simulink library "r2daq_blocks"  (R2012b)
settings: Solver=ode45  StartTime=0.0  StopTime=10.0  RelTol=1e-3
undefined symbols (not defined in the file or in its folder): biquad_iir, feedback_iir, filters, libddc, sfp, synth, xlfir_8x16
libraries: xbsIndex_r4 x4088, casper_library_misc x21, dspsigops x16, casper_library_delays x10, xps_library x1
(part 5 of 23)

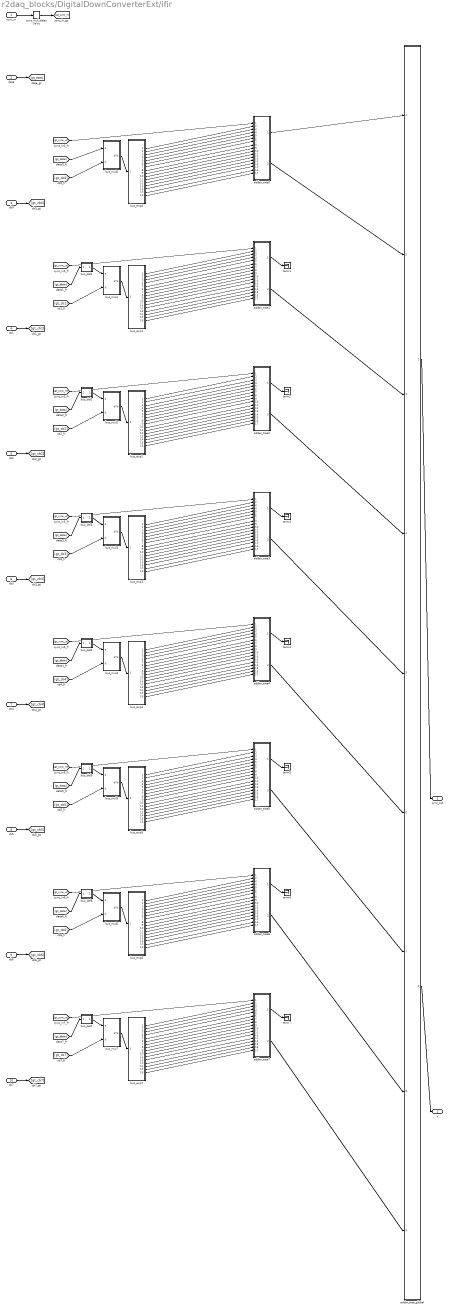
== system r2daq_blocks/DigitalDownConverterExt/ifir ==
  sync_in : Inport
  data : Inport  Port=2
  cb0 : Inport  Port=3
  cb1 : Inport  Port=4
  cb2 : Inport  Port=5
  cb3 : Inport  Port=6
  cb4 : Inport  Port=7
  cb5 : Inport  Port=8
  cb6 : Inport  Port=9
  cb7 : Inport  Port=10
  adder_tree0 : Subsystem  AncestorBlock=casper_library_misc/adder_tree  mask(adder_tree){n_inputs=16, latency=1, adder_imp=Fabric, first_stage_hdl=on}
      mask prompts: n_inputs "Number of Inputs"; latency "Add Latency"; adder_imp "Adder implementation"; first_stage_hdl "Use behavioural HDL for first stage of adders"
      mask help:
      | Sums all inputs using a tree of adds and delays.
      |
      | Number of inputs: The number of inputs to the block to be summed
      | Add latency: The number of clock cycles to perform one addition (affects timing)..
      | Adder implementation: choice of fabric or DSP48E core, or behavioral HDL
      | Use behavioural HDL for first stage of adders: Causes the first stage of adders to be absorbed into DSP blocks if multipliers precede them (Virtex 5). Overrides Adder implementation
      mask init:
      | adder_tree_init(gcb, ...
      |     'n_inputs', n_inputs, ...
      |     'latency', latency, ...
      |     'adder_imp', adder_imp, ...
      |     'first_stage_hdl', first_stage_hdl);
      settings: AttributesFormatString=latency 4
      mask Help: eval('xlWeb(''http://casper.berkeley.edu/wiki/Adder_tree'')')
      mask TypeOptions adder_imp: Behavioral | Fabric | DSP48
  adder_tree1 : Subsystem  AncestorBlock=casper_library_misc/adder_tree  mask(adder_tree){n_inputs=16, latency=1, adder_imp=Fabric, first_stage_hdl=on}
      mask prompts: n_inputs "Number of Inputs"; latency "Add Latency"; adder_imp "Adder implementation"; first_stage_hdl "Use behavioural HDL for first stage of adders"
      mask help:
      | Sums all inputs using a tree of adds and delays.
      |
      | Number of inputs: The number of inputs to the block to be summed
      | Add latency: The number of clock cycles to perform one addition (affects timing)..
      | Adder implementation: choice of fabric or DSP48E core, or behavioral HDL
      | Use behavioural HDL for first stage of adders: Causes the first stage of adders to be absorbed into DSP blocks if multipliers precede them (Virtex 5). Overrides Adder implementation
      mask init:
      | adder_tree_init(gcb, ...
      |     'n_inputs', n_inputs, ...
      |     'latency', latency, ...
      |     'adder_imp', adder_imp, ...
      |     'first_stage_hdl', first_stage_hdl);
      settings: AttributesFormatString=latency 4
      mask Help: eval('xlWeb(''http://casper.berkeley.edu/wiki/Adder_tree'')')
      mask TypeOptions adder_imp: Behavioral | Fabric | DSP48
  adder_tree2 : Subsystem  AncestorBlock=casper_library_misc/adder_tree  mask(adder_tree){n_inputs=16, latency=1, adder_imp=Fabric, first_stage_hdl=on}
      mask prompts: n_inputs "Number of Inputs"; latency "Add Latency"; adder_imp "Adder implementation"; first_stage_hdl "Use behavioural HDL for first stage of adders"
      mask help:
      | Sums all inputs using a tree of adds and delays.
      |
      | Number of inputs: The number of inputs to the block to be summed
      | Add latency: The number of clock cycles to perform one addition (affects timing)..
      | Adder implementation: choice of fabric or DSP48E core, or behavioral HDL
      | Use behavioural HDL for first stage of adders: Causes the first stage of adders to be absorbed into DSP blocks if multipliers precede them (Virtex 5). Overrides Adder implementation
      mask init:
      | adder_tree_init(gcb, ...
      |     'n_inputs', n_inputs, ...
      |     'latency', latency, ...
      |     'adder_imp', adder_imp, ...
      |     'first_stage_hdl', first_stage_hdl);
      settings: AttributesFormatString=latency 4
      mask Help: eval('xlWeb(''http://casper.berkeley.edu/wiki/Adder_tree'')')
      mask TypeOptions adder_imp: Behavioral | Fabric | DSP48
  adder_tree3 : Subsystem  AncestorBlock=casper_library_misc/adder_tree  mask(adder_tree){n_inputs=16, latency=1, adder_imp=Fabric, first_stage_hdl=on}
      mask prompts: n_inputs "Number of Inputs"; latency "Add Latency"; adder_imp "Adder implementation"; first_stage_hdl "Use behavioural HDL for first stage of adders"
      mask help:
      | Sums all inputs using a tree of adds and delays.
      |
      | Number of inputs: The number of inputs to the block to be summed
      | Add latency: The number of clock cycles to perform one addition (affects timing)..
      | Adder implementation: choice of fabric or DSP48E core, or behavioral HDL
      | Use behavioural HDL for first stage of adders: Causes the first stage of adders to be absorbed into DSP blocks if multipliers precede them (Virtex 5). Overrides Adder implementation
      mask init:
      | adder_tree_init(gcb, ...
      |     'n_inputs', n_inputs, ...
      |     'latency', latency, ...
      |     'adder_imp', adder_imp, ...
      |     'first_stage_hdl', first_stage_hdl);
      settings: AttributesFormatString=latency 4
      mask Help: eval('xlWeb(''http://casper.berkeley.edu/wiki/Adder_tree'')')
      mask TypeOptions adder_imp: Behavioral | Fabric | DSP48
  adder_tree4 : Subsystem  AncestorBlock=casper_library_misc/adder_tree  mask(adder_tree){n_inputs=16, latency=1, adder_imp=Fabric, first_stage_hdl=on}
      mask prompts: n_inputs "Number of Inputs"; latency "Add Latency"; adder_imp "Adder implementation"; first_stage_hdl "Use behavioural HDL for first stage of adders"
      mask help:
      | Sums all inputs using a tree of adds and delays.
      |
      | Number of inputs: The number of inputs to the block to be summed
      | Add latency: The number of clock cycles to perform one addition (affects timing)..
      | Adder implementation: choice of fabric or DSP48E core, or behavioral HDL
      | Use behavioural HDL for first stage of adders: Causes the first stage of adders to be absorbed into DSP blocks if multipliers precede them (Virtex 5). Overrides Adder implementation
      mask init:
      | adder_tree_init(gcb, ...
      |     'n_inputs', n_inputs, ...
      |     'latency', latency, ...
      |     'adder_imp', adder_imp, ...
      |     'first_stage_hdl', first_stage_hdl);
      settings: AttributesFormatString=latency 4
      mask Help: eval('xlWeb(''http://casper.berkeley.edu/wiki/Adder_tree'')')
      mask TypeOptions adder_imp: Behavioral | Fabric | DSP48
  adder_tree5 : Subsystem  AncestorBlock=casper_library_misc/adder_tree  mask(adder_tree){n_inputs=16, latency=1, adder_imp=Fabric, first_stage_hdl=on}
      mask prompts: n_inputs "Number of Inputs"; latency "Add Latency"; adder_imp "Adder implementation"; first_stage_hdl "Use behavioural HDL for first stage of adders"
      mask help:
      | Sums all inputs using a tree of adds and delays.
      |
      | Number of inputs: The number of inputs to the block to be summed
      | Add latency: The number of clock cycles to perform one addition (affects timing)..
      | Adder implementation: choice of fabric or DSP48E core, or behavioral HDL
      | Use behavioural HDL for first stage of adders: Causes the first stage of adders to be absorbed into DSP blocks if multipliers precede them (Virtex 5). Overrides Adder implementation
      mask init:
      | adder_tree_init(gcb, ...
      |     'n_inputs', n_inputs, ...
      |     'latency', latency, ...
      |     'adder_imp', adder_imp, ...
      |     'first_stage_hdl', first_stage_hdl);
      settings: AttributesFormatString=latency 4
      mask Help: eval('xlWeb(''http://casper.berkeley.edu/wiki/Adder_tree'')')
      mask TypeOptions adder_imp: Behavioral | Fabric | DSP48
  adder_tree6 : Subsystem  AncestorBlock=casper_library_misc/adder_tree  mask(adder_tree){n_inputs=16, latency=1, adder_imp=Fabric, first_stage_hdl=on}
      mask prompts: n_inputs "Number of Inputs"; latency "Add Latency"; adder_imp "Adder implementation"; first_stage_hdl "Use behavioural HDL for first stage of adders"
      mask help:
      | Sums all inputs using a tree of adds and delays.
      |
      | Number of inputs: The number of inputs to the block to be summed
      | Add latency: The number of clock cycles to perform one addition (affects timing)..
      | Adder implementation: choice of fabric or DSP48E core, or behavioral HDL
      | Use behavioural HDL for first stage of adders: Causes the first stage of adders to be absorbed into DSP blocks if multipliers precede them (Virtex 5). Overrides Adder implementation
      mask init:
      | adder_tree_init(gcb, ...
      |     'n_inputs', n_inputs, ...
      |     'latency', latency, ...
      |     'adder_imp', adder_imp, ...
      |     'first_stage_hdl', first_stage_hdl);
      settings: AttributesFormatString=latency 4
      mask Help: eval('xlWeb(''http://casper.berkeley.edu/wiki/Adder_tree'')')
      mask TypeOptions adder_imp: Behavioral | Fabric | DSP48
  adder_tree7 : Subsystem  AncestorBlock=casper_library_misc/adder_tree  mask(adder_tree){n_inputs=16, latency=1, adder_imp=Fabric, first_stage_hdl=on}
      mask prompts: n_inputs "Number of Inputs"; latency "Add Latency"; adder_imp "Adder implementation"; first_stage_hdl "Use behavioural HDL for first stage of adders"
      mask help:
      | Sums all inputs using a tree of adds and delays.
      |
      | Number of inputs: The number of inputs to the block to be summed
      | Add latency: The number of clock cycles to perform one addition (affects timing)..
      | Adder implementation: choice of fabric or DSP48E core, or behavioral HDL
      | Use behavioural HDL for first stage of adders: Causes the first stage of adders to be absorbed into DSP blocks if multipliers precede them (Virtex 5). Overrides Adder implementation
      mask init:
      | adder_tree_init(gcb, ...
      |     'n_inputs', n_inputs, ...
      |     'latency', latency, ...
      |     'adder_imp', adder_imp, ...
      |     'first_stage_hdl', first_stage_hdl);
      settings: AttributesFormatString=latency 4
      mask Help: eval('xlWeb(''http://casper.berkeley.edu/wiki/Adder_tree'')')
      mask TypeOptions adder_imp: Behavioral | Fabric | DSP48
  adder_tree_global : Subsystem  AncestorBlock=casper_library_misc/adder_tree  mask(adder_tree){n_inputs=8, latency=1, adder_imp=Fabric, first_stage_hdl=on}
      mask prompts: n_inputs "Number of Inputs"; latency "Add Latency"; adder_imp "Adder implementation"; first_stage_hdl "Use behavioural HDL for first stage of adders"
      mask help:
      | Sums all inputs using a tree of adds and delays.
      |
      | Number of inputs: The number of inputs to the block to be summed
      | Add latency: The number of clock cycles to perform one addition (affects timing)..
      | Adder implementation: choice of fabric or DSP48E core, or behavioral HDL
      | Use behavioural HDL for first stage of adders: Causes the first stage of adders to be absorbed into DSP blocks if multipliers precede them (Virtex 5). Overrides Adder implementation
      mask init:
      | adder_tree_init(gcb, ...
      |     'n_inputs', n_inputs, ...
      |     'latency', latency, ...
      |     'adder_imp', adder_imp, ...
      |     'first_stage_hdl', first_stage_hdl);
      settings: AttributesFormatString=latency 3
      mask Help: eval('xlWeb(''http://casper.berkeley.edu/wiki/Adder_tree'')')
      mask TypeOptions adder_imp: Behavioral | Fabric | DSP48
  bus_del1 : Subsystem  AncestorBlock=casper_library_bus/bus_delay  mask(bus_delay){n_bits=[18 18 18 18 18 18 18 18 18 18 18 18 18 18 18 18], latency=1, cmplx=off, enable=off, reg_retiming=on, misc=off}
      mask prompts: n_bits "input bit widths"; cmplx "complex data"; enable "enable port"; reg_retiming "implement using behavioral HDL"; misc "misc support"
      mask help: Delay components of a bus
      mask init:
      | bus_delay_init(gcb, ...
      |     'enable', enable, ...
      |     'cmplx', cmplx, ...
      |     'n_bits', n_bits, ...
      |     'latency', latency, ...
      |     'reg_retiming', reg_retiming, ...
      |     'misc', misc);
  bus_del2 : Subsystem  AncestorBlock=casper_library_bus/bus_delay  mask(bus_delay){n_bits=[18 18 18 18 18 18 18 18 18 18 18 18 18 18 18 18], latency=2, cmplx=off, enable=off, reg_retiming=on, misc=off}
      mask prompts: n_bits "input bit widths"; cmplx "complex data"; enable "enable port"; reg_retiming "implement using behavioral HDL"; misc "misc support"
      mask help: Delay components of a bus
      mask init:
      | bus_delay_init(gcb, ...
      |     'enable', enable, ...
      |     'cmplx', cmplx, ...
      |     'n_bits', n_bits, ...
      |     'latency', latency, ...
      |     'reg_retiming', reg_retiming, ...
      |     'misc', misc);
  bus_del3 : Subsystem  AncestorBlock=casper_library_bus/bus_delay  mask(bus_delay){n_bits=[18 18 18 18 18 18 18 18 18 18 18 18 18 18 18 18], latency=3, cmplx=off, enable=off, reg_retiming=on, misc=off}
      mask prompts: n_bits "input bit widths"; cmplx "complex data"; enable "enable port"; reg_retiming "implement using behavioral HDL"; misc "misc support"
      mask help: Delay components of a bus
      mask init:
      | bus_delay_init(gcb, ...
      |     'enable', enable, ...
      |     'cmplx', cmplx, ...
      |     'n_bits', n_bits, ...
      |     'latency', latency, ...
      |     'reg_retiming', reg_retiming, ...
      |     'misc', misc);
  bus_del4 : Subsystem  AncestorBlock=casper_library_bus/bus_delay  mask(bus_delay){n_bits=[18 18 18 18 18 18 18 18 18 18 18 18 18 18 18 18], latency=4, cmplx=off, enable=off, reg_retiming=on, misc=off}
      mask prompts: n_bits "input bit widths"; cmplx "complex data"; enable "enable port"; reg_retiming "implement using behavioral HDL"; misc "misc support"
      mask help: Delay components of a bus
      mask init:
      | bus_delay_init(gcb, ...
      |     'enable', enable, ...
      |     'cmplx', cmplx, ...
      |     'n_bits', n_bits, ...
      |     'latency', latency, ...
      |     'reg_retiming', reg_retiming, ...
      |     'misc', misc);
  bus_del5 : Subsystem  AncestorBlock=casper_library_bus/bus_delay  mask(bus_delay){n_bits=[18 18 18 18 18 18 18 18 18 18 18 18 18 18 18 18], latency=5, cmplx=off, enable=off, reg_retiming=on, misc=off}
      mask prompts: n_bits "input bit widths"; cmplx "complex data"; enable "enable port"; reg_retiming "implement using behavioral HDL"; misc "misc support"
      mask help: Delay components of a bus
      mask init:
      | bus_delay_init(gcb, ...
      |     'enable', enable, ...
      |     'cmplx', cmplx, ...
      |     'n_bits', n_bits, ...
      |     'latency', latency, ...
      |     'reg_retiming', reg_retiming, ...
      |     'misc', misc);
  bus_del6 : Subsystem  AncestorBlock=casper_library_bus/bus_delay  mask(bus_delay){n_bits=[18 18 18 18 18 18 18 18 18 18 18 18 18 18 18 18], latency=6, cmplx=off, enable=off, reg_retiming=on, misc=off}
      mask prompts: n_bits "input bit widths"; cmplx "complex data"; enable "enable port"; reg_retiming "implement using behavioral HDL"; misc "misc support"
      mask help: Delay components of a bus
      mask init:
      | bus_delay_init(gcb, ...
      |     'enable', enable, ...
      |     'cmplx', cmplx, ...
      |     'n_bits', n_bits, ...
      |     'latency', latency, ...
      |     'reg_retiming', reg_retiming, ...
      |     'misc', misc);
  bus_del7 : Subsystem  AncestorBlock=casper_library_bus/bus_delay  mask(bus_delay){n_bits=[18 18 18 18 18 18 18 18 18 18 18 18 18 18 18 18], latency=7, cmplx=off, enable=off, reg_retiming=on, misc=off}
      mask prompts: n_bits "input bit widths"; cmplx "complex data"; enable "enable port"; reg_retiming "implement using behavioral HDL"; misc "misc support"
      mask help: Delay components of a bus
      mask init:
      | bus_delay_init(gcb, ...
      |     'enable', enable, ...
      |     'cmplx', cmplx, ...
      |     'n_bits', n_bits, ...
      |     'latency', latency, ...
      |     'reg_retiming', reg_retiming, ...
      |     'misc', misc);
  bus_exp0 : Subsystem  AncestorBlock=casper_library_flow_control/bus_expand  mask(bus_expand){mode=divisions of equal size, outputNum=16, outputWidth=18, outputBinaryPt=16, outputArithmeticType=1, show_format=off, outputToWorkspace=off, variablePrefix=out, outputToModelAsWell=on}
      mask prompts: outputNum "Number of outputs:"; outputWidth "Output width:"; outputBinaryPt "Output binary point position:"; outputArithmeticType "Output arithmetic type (ufix=0, fix=1, bool=2):"; show_format "Print format string?"; outputToWorkspace "Output to workspace?"; variablePrefix "Variable name prefix:"; outputToModelAsWell "Output to model as well?"
      mask help:
      | Expands a 'bus' made using a bus_create or Xilinx
      | concat block.
      | The input will be divided into the specified number
      | of outputs with the specified arithmetic types.
      | Divisions are made from most significant bit.
      mask init: same as r2daq_blocks/DigitalDownConverterExt/bus_mul_cosine/a_debus
      settings: AttributesFormatString=16 outputs
      mask TypeOptions mode: divisions of equal size | divisions of arbitrary size
      mask Callback mode: bus_expand_callback();
      mask Callback outputWidth: bus_expand_callback();
      mask Callback outputToWorkspace: bus_expand_callback();
  bus_exp1 : Subsystem  AncestorBlock=casper_library_flow_control/bus_expand  mask(bus_expand){mode=divisions of equal size, outputNum=16, outputWidth=18, outputBinaryPt=16, outputArithmeticType=1, show_format=off, outputToWorkspace=off, variablePrefix=out, outputToModelAsWell=on}
      mask prompts: outputNum "Number of outputs:"; outputWidth "Output width:"; outputBinaryPt "Output binary point position:"; outputArithmeticType "Output arithmetic type (ufix=0, fix=1, bool=2):"; show_format "Print format string?"; outputToWorkspace "Output to workspace?"; variablePrefix "Variable name prefix:"; outputToModelAsWell "Output to model as well?"
      mask help:
      | Expands a 'bus' made using a bus_create or Xilinx
      | concat block.
      | The input will be divided into the specified number
      | of outputs with the specified arithmetic types.
      | Divisions are made from most significant bit.
      mask init: same as r2daq_blocks/DigitalDownConverterExt/bus_mul_cosine/a_debus
      settings: AttributesFormatString=16 outputs
      mask TypeOptions mode: divisions of equal size | divisions of arbitrary size
      mask Callback mode: bus_expand_callback();
      mask Callback outputWidth: bus_expand_callback();
      mask Callback outputToWorkspace: bus_expand_callback();
  bus_exp2 : Subsystem  AncestorBlock=casper_library_flow_control/bus_expand  mask(bus_expand){mode=divisions of equal size, outputNum=16, outputWidth=18, outputBinaryPt=16, outputArithmeticType=1, show_format=off, outputToWorkspace=off, variablePrefix=out, outputToModelAsWell=on}
      mask prompts: outputNum "Number of outputs:"; outputWidth "Output width:"; outputBinaryPt "Output binary point position:"; outputArithmeticType "Output arithmetic type (ufix=0, fix=1, bool=2):"; show_format "Print format string?"; outputToWorkspace "Output to workspace?"; variablePrefix "Variable name prefix:"; outputToModelAsWell "Output to model as well?"
      mask help:
      | Expands a 'bus' made using a bus_create or Xilinx
      | concat block.
      | The input will be divided into the specified number
      | of outputs with the specified arithmetic types.
      | Divisions are made from most significant bit.
      mask init: same as r2daq_blocks/DigitalDownConverterExt/bus_mul_cosine/a_debus
      settings: AttributesFormatString=16 outputs
      mask TypeOptions mode: divisions of equal size | divisions of arbitrary size
      mask Callback mode: bus_expand_callback();
      mask Callback outputWidth: bus_expand_callback();
      mask Callback outputToWorkspace: bus_expand_callback();
  bus_exp3 : Subsystem  AncestorBlock=casper_library_flow_control/bus_expand  mask(bus_expand){mode=divisions of equal size, outputNum=16, outputWidth=18, outputBinaryPt=16, outputArithmeticType=1, show_format=off, outputToWorkspace=off, variablePrefix=out, outputToModelAsWell=on}
      mask prompts: outputNum "Number of outputs:"; outputWidth "Output width:"; outputBinaryPt "Output binary point position:"; outputArithmeticType "Output arithmetic type (ufix=0, fix=1, bool=2):"; show_format "Print format string?"; outputToWorkspace "Output to workspace?"; variablePrefix "Variable name prefix:"; outputToModelAsWell "Output to model as well?"
      mask help:
      | Expands a 'bus' made using a bus_create or Xilinx
      | concat block.
      | The input will be divided into the specified number
      | of outputs with the specified arithmetic types.
      | Divisions are made from most significant bit.
      mask init: same as r2daq_blocks/DigitalDownConverterExt/bus_mul_cosine/a_debus
      settings: AttributesFormatString=16 outputs
      mask TypeOptions mode: divisions of equal size | divisions of arbitrary size
      mask Callback mode: bus_expand_callback();
      mask Callback outputWidth: bus_expand_callback();
      mask Callback outputToWorkspace: bus_expand_callback();
  bus_exp4 : Subsystem  AncestorBlock=casper_library_flow_control/bus_expand  mask(bus_expand){mode=divisions of equal size, outputNum=16, outputWidth=18, outputBinaryPt=16, outputArithmeticType=1, show_format=off, outputToWorkspace=off, variablePrefix=out, outputToModelAsWell=on}
      mask prompts: outputNum "Number of outputs:"; outputWidth "Output width:"; outputBinaryPt "Output binary point position:"; outputArithmeticType "Output arithmetic type (ufix=0, fix=1, bool=2):"; show_format "Print format string?"; outputToWorkspace "Output to workspace?"; variablePrefix "Variable name prefix:"; outputToModelAsWell "Output to model as well?"
      mask help:
      | Expands a 'bus' made using a bus_create or Xilinx
      | concat block.
      | The input will be divided into the specified number
      | of outputs with the specified arithmetic types.
      | Divisions are made from most significant bit.
      mask init: same as r2daq_blocks/DigitalDownConverterExt/bus_mul_cosine/a_debus
      settings: AttributesFormatString=16 outputs
      mask TypeOptions mode: divisions of equal size | divisions of arbitrary size
      mask Callback mode: bus_expand_callback();
      mask Callback outputWidth: bus_expand_callback();
      mask Callback outputToWorkspace: bus_expand_callback();
  bus_exp5 : Subsystem  AncestorBlock=casper_library_flow_control/bus_expand  mask(bus_expand){mode=divisions of equal size, outputNum=16, outputWidth=18, outputBinaryPt=16, outputArithmeticType=1, show_format=off, outputToWorkspace=off, variablePrefix=out, outputToModelAsWell=on}
      mask prompts: outputNum "Number of outputs:"; outputWidth "Output width:"; outputBinaryPt "Output binary point position:"; outputArithmeticType "Output arithmetic type (ufix=0, fix=1, bool=2):"; show_format "Print format string?"; outputToWorkspace "Output to workspace?"; variablePrefix "Variable name prefix:"; outputToModelAsWell "Output to model as well?"
      mask help:
      | Expands a 'bus' made using a bus_create or Xilinx
      | concat block.
      | The input will be divided into the specified number
      | of outputs with the specified arithmetic types.
      | Divisions are made from most significant bit.
      mask init: same as r2daq_blocks/DigitalDownConverterExt/bus_mul_cosine/a_debus
      settings: AttributesFormatString=16 outputs
      mask TypeOptions mode: divisions of equal size | divisions of arbitrary size
      mask Callback mode: bus_expand_callback();
      mask Callback outputWidth: bus_expand_callback();
      mask Callback outputToWorkspace: bus_expand_callback();
  bus_exp6 : Subsystem  AncestorBlock=casper_library_flow_control/bus_expand  mask(bus_expand){mode=divisions of equal size, outputNum=16, outputWidth=18, outputBinaryPt=16, outputArithmeticType=1, show_format=off, outputToWorkspace=off, variablePrefix=out, outputToModelAsWell=on}
      mask prompts: outputNum "Number of outputs:"; outputWidth "Output width:"; outputBinaryPt "Output binary point position:"; outputArithmeticType "Output arithmetic type (ufix=0, fix=1, bool=2):"; show_format "Print format string?"; outputToWorkspace "Output to workspace?"; variablePrefix "Variable name prefix:"; outputToModelAsWell "Output to model as well?"
      mask help:
      | Expands a 'bus' made using a bus_create or Xilinx
      | concat block.
      | The input will be divided into the specified number
      | of outputs with the specified arithmetic types.
      | Divisions are made from most significant bit.
      mask init: same as r2daq_blocks/DigitalDownConverterExt/bus_mul_cosine/a_debus
      settings: AttributesFormatString=16 outputs
      mask TypeOptions mode: divisions of equal size | divisions of arbitrary size
      mask Callback mode: bus_expand_callback();
      mask Callback outputWidth: bus_expand_callback();
      mask Callback outputToWorkspace: bus_expand_callback();
  bus_exp7 : Subsystem  AncestorBlock=casper_library_flow_control/bus_expand  mask(bus_expand){mode=divisions of equal size, outputNum=16, outputWidth=18, outputBinaryPt=16, outputArithmeticType=1, show_format=off, outputToWorkspace=off, variablePrefix=out, outputToModelAsWell=on}
      mask prompts: outputNum "Number of outputs:"; outputWidth "Output width:"; outputBinaryPt "Output binary point position:"; outputArithmeticType "Output arithmetic type (ufix=0, fix=1, bool=2):"; show_format "Print format string?"; outputToWorkspace "Output to workspace?"; variablePrefix "Variable name prefix:"; outputToModelAsWell "Output to model as well?"
      mask help:
      | Expands a 'bus' made using a bus_create or Xilinx
      | concat block.
      | The input will be divided into the specified number
      | of outputs with the specified arithmetic types.
      | Divisions are made from most significant bit.
      mask init: same as r2daq_blocks/DigitalDownConverterExt/bus_mul_cosine/a_debus
      settings: AttributesFormatString=16 outputs
      mask TypeOptions mode: divisions of equal size | divisions of arbitrary size
      mask Callback mode: bus_expand_callback();
      mask Callback outputWidth: bus_expand_callback();
      mask Callback outputToWorkspace: bus_expand_callback();
  bus_mul0 : Subsystem  AncestorBlock=casper_library_bus/bus_mult  mask(bus_mult){n_bits_a=[18 18 18 18 18 18 18 18 18 18 18 18 18 18 18 18], bin_pt_a=[16 16 16 16 16 16 16 16 16 16 16 16 16 16 16 16], type_a=[1 1 1 1 1 1 1 1 1 1 1 1 1 1 1 1], cmplx_a=off, n_bits_b=[8 8 8 8 8 8 8 8 8 8 8 8 8 8 8 8], bin_pt_b=[7 7 7 7 7 7 7 7 7 7 7 7 7 7 7 7], type_b=[1 1 1 1 1 1 1 1 1 1 1 1 1 1 1 1], cmplx_b=off, n_bits_out=[18 18 18 18 18 18 18 18 18 18 18 18 18 18 18 18], bin_pt_out=[16 16 16 16 16 16 16 16 16 16 16 16 16 16 16 16], type_out=[1 1 1 1 1 1 1 1 1 1 1 1 1 1 1 1], quantization=0, overflow=0, mult_latency=3, add_latency=1, conv_latency=1, max_fanout=2, fan_latency=0, multiplier_implementation=behavioral HDL, misc=off}
      mask prompts: n_bits_a "a input bit widths"; bin_pt_a "a input binary points"; type_a "a input type (Unsigned=0, Signed=1)"; cmplx_a "a input complex"; n_bits_b "b input bit widths"; bin_pt_b "b input binary points"; type_b "b input type (Unsigned=0, Signed=1)"; cmplx_b "b input complex"; n_bits_out "output bit widths"; bin_pt_out "output binary points"; type_out "output type (Unsigned=0, Signed=1)"; quantization "quantization strategy (Truncate=0, Round  (unbiased: +/- Inf)=1)"; overflow "overflow strategy (Wrap=0, Saturate=1, Flag as error=2)"; mult_latency "multiplier latency"; add_latency "adder latency"; conv_latency "convert latency"; max_fanout "limit fanout to ?"; fan_latency "fanout register latency"; multiplier_implementation "multiplier implementation"; misc "misc support"
      mask help: Multiply components of two busses
      mask init: same as r2daq_blocks/DigitalDownConverterExt/bus_mul_cosine
      mask TypeOptions multiplier_implementation: behavioral HDL | standard core | embedded multiplier core
  bus_mul1 : Subsystem  AncestorBlock=casper_library_bus/bus_mult  mask(bus_mult){n_bits_a=[18 18 18 18 18 18 18 18 18 18 18 18 18 18 18 18], bin_pt_a=[16 16 16 16 16 16 16 16 16 16 16 16 16 16 16 16], type_a=[1 1 1 1 1 1 1 1 1 1 1 1 1 1 1 1], cmplx_a=off, n_bits_b=[8 8 8 8 8 8 8 8 8 8 8 8 8 8 8 8], bin_pt_b=[7 7 7 7 7 7 7 7 7 7 7 7 7 7 7 7], type_b=[1 1 1 1 1 1 1 1 1 1 1 1 1 1 1 1], cmplx_b=off, n_bits_out=[18 18 18 18 18 18 18 18 18 18 18 18 18 18 18 18], bin_pt_out=[16 16 16 16 16 16 16 16 16 16 16 16 16 16 16 16], type_out=[1 1 1 1 1 1 1 1 1 1 1 1 1 1 1 1], quantization=0, overflow=0, mult_latency=3, add_latency=1, conv_latency=1, max_fanout=2, fan_latency=0, multiplier_implementation=behavioral HDL, misc=off}
      mask prompts: n_bits_a "a input bit widths"; bin_pt_a "a input binary points"; type_a "a input type (Unsigned=0, Signed=1)"; cmplx_a "a input complex"; n_bits_b "b input bit widths"; bin_pt_b "b input binary points"; type_b "b input type (Unsigned=0, Signed=1)"; cmplx_b "b input complex"; n_bits_out "output bit widths"; bin_pt_out "output binary points"; type_out "output type (Unsigned=0, Signed=1)"; quantization "quantization strategy (Truncate=0, Round  (unbiased: +/- Inf)=1)"; overflow "overflow strategy (Wrap=0, Saturate=1, Flag as error=2)"; mult_latency "multiplier latency"; add_latency "adder latency"; conv_latency "convert latency"; max_fanout "limit fanout to ?"; fan_latency "fanout register latency"; multiplier_implementation "multiplier implementation"; misc "misc support"
      mask help: Multiply components of two busses
      mask init: same as r2daq_blocks/DigitalDownConverterExt/bus_mul_cosine
      mask TypeOptions multiplier_implementation: behavioral HDL | standard core | embedded multiplier core
  bus_mul2 : Subsystem  AncestorBlock=casper_library_bus/bus_mult  mask(bus_mult){n_bits_a=[18 18 18 18 18 18 18 18 18 18 18 18 18 18 18 18], bin_pt_a=[16 16 16 16 16 16 16 16 16 16 16 16 16 16 16 16], type_a=[1 1 1 1 1 1 1 1 1 1 1 1 1 1 1 1], cmplx_a=off, n_bits_b=[8 8 8 8 8 8 8 8 8 8 8 8 8 8 8 8], bin_pt_b=[7 7 7 7 7 7 7 7 7 7 7 7 7 7 7 7], type_b=[1 1 1 1 1 1 1 1 1 1 1 1 1 1 1 1], cmplx_b=off, n_bits_out=[18 18 18 18 18 18 18 18 18 18 18 18 18 18 18 18], bin_pt_out=[16 16 16 16 16 16 16 16 16 16 16 16 16 16 16 16], type_out=[1 1 1 1 1 1 1 1 1 1 1 1 1 1 1 1], quantization=0, overflow=0, mult_latency=3, add_latency=1, conv_latency=1, max_fanout=2, fan_latency=0, multiplier_implementation=behavioral HDL, misc=off}
      mask prompts: n_bits_a "a input bit widths"; bin_pt_a "a input binary points"; type_a "a input type (Unsigned=0, Signed=1)"; cmplx_a "a input complex"; n_bits_b "b input bit widths"; bin_pt_b "b input binary points"; type_b "b input type (Unsigned=0, Signed=1)"; cmplx_b "b input complex"; n_bits_out "output bit widths"; bin_pt_out "output binary points"; type_out "output type (Unsigned=0, Signed=1)"; quantization "quantization strategy (Truncate=0, Round  (unbiased: +/- Inf)=1)"; overflow "overflow strategy (Wrap=0, Saturate=1, Flag as error=2)"; mult_latency "multiplier latency"; add_latency "adder latency"; conv_latency "convert latency"; max_fanout "limit fanout to ?"; fan_latency "fanout register latency"; multiplier_implementation "multiplier implementation"; misc "misc support"
      mask help: Multiply components of two busses
      mask init: same as r2daq_blocks/DigitalDownConverterExt/bus_mul_cosine
      mask TypeOptions multiplier_implementation: behavioral HDL | standard core | embedded multiplier core
  bus_mul3 : Subsystem  AncestorBlock=casper_library_bus/bus_mult  mask(bus_mult){n_bits_a=[18 18 18 18 18 18 18 18 18 18 18 18 18 18 18 18], bin_pt_a=[16 16 16 16 16 16 16 16 16 16 16 16 16 16 16 16], type_a=[1 1 1 1 1 1 1 1 1 1 1 1 1 1 1 1], cmplx_a=off, n_bits_b=[8 8 8 8 8 8 8 8 8 8 8 8 8 8 8 8], bin_pt_b=[7 7 7 7 7 7 7 7 7 7 7 7 7 7 7 7], type_b=[1 1 1 1 1 1 1 1 1 1 1 1 1 1 1 1], cmplx_b=off, n_bits_out=[18 18 18 18 18 18 18 18 18 18 18 18 18 18 18 18], bin_pt_out=[16 16 16 16 16 16 16 16 16 16 16 16 16 16 16 16], type_out=[1 1 1 1 1 1 1 1 1 1 1 1 1 1 1 1], quantization=0, overflow=0, mult_latency=3, add_latency=1, conv_latency=1, max_fanout=2, fan_latency=0, multiplier_implementation=behavioral HDL, misc=off}
      mask prompts: n_bits_a "a input bit widths"; bin_pt_a "a input binary points"; type_a "a input type (Unsigned=0, Signed=1)"; cmplx_a "a input complex"; n_bits_b "b input bit widths"; bin_pt_b "b input binary points"; type_b "b input type (Unsigned=0, Signed=1)"; cmplx_b "b input complex"; n_bits_out "output bit widths"; bin_pt_out "output binary points"; type_out "output type (Unsigned=0, Signed=1)"; quantization "quantization strategy (Truncate=0, Round  (unbiased: +/- Inf)=1)"; overflow "overflow strategy (Wrap=0, Saturate=1, Flag as error=2)"; mult_latency "multiplier latency"; add_latency "adder latency"; conv_latency "convert latency"; max_fanout "limit fanout to ?"; fan_latency "fanout register latency"; multiplier_implementation "multiplier implementation"; misc "misc support"
      mask help: Multiply components of two busses
      mask init: same as r2daq_blocks/DigitalDownConverterExt/bus_mul_cosine
      mask TypeOptions multiplier_implementation: behavioral HDL | standard core | embedded multiplier core
  bus_mul4 : Subsystem  AncestorBlock=casper_library_bus/bus_mult  mask(bus_mult){n_bits_a=[18 18 18 18 18 18 18 18 18 18 18 18 18 18 18 18], bin_pt_a=[16 16 16 16 16 16 16 16 16 16 16 16 16 16 16 16], type_a=[1 1 1 1 1 1 1 1 1 1 1 1 1 1 1 1], cmplx_a=off, n_bits_b=[8 8 8 8 8 8 8 8 8 8 8 8 8 8 8 8], bin_pt_b=[7 7 7 7 7 7 7 7 7 7 7 7 7 7 7 7], type_b=[1 1 1 1 1 1 1 1 1 1 1 1 1 1 1 1], cmplx_b=off, n_bits_out=[18 18 18 18 18 18 18 18 18 18 18 18 18 18 18 18], bin_pt_out=[16 16 16 16 16 16 16 16 16 16 16 16 16 16 16 16], type_out=[1 1 1 1 1 1 1 1 1 1 1 1 1 1 1 1], quantization=0, overflow=0, mult_latency=3, add_latency=1, conv_latency=1, max_fanout=2, fan_latency=0, multiplier_implementation=behavioral HDL, misc=off}
      mask prompts: n_bits_a "a input bit widths"; bin_pt_a "a input binary points"; type_a "a input type (Unsigned=0, Signed=1)"; cmplx_a "a input complex"; n_bits_b "b input bit widths"; bin_pt_b "b input binary points"; type_b "b input type (Unsigned=0, Signed=1)"; cmplx_b "b input complex"; n_bits_out "output bit widths"; bin_pt_out "output binary points"; type_out "output type (Unsigned=0, Signed=1)"; quantization "quantization strategy (Truncate=0, Round  (unbiased: +/- Inf)=1)"; overflow "overflow strategy (Wrap=0, Saturate=1, Flag as error=2)"; mult_latency "multiplier latency"; add_latency "adder latency"; conv_latency "convert latency"; max_fanout "limit fanout to ?"; fan_latency "fanout register latency"; multiplier_implementation "multiplier implementation"; misc "misc support"
      mask help: Multiply components of two busses
      mask init: same as r2daq_blocks/DigitalDownConverterExt/bus_mul_cosine
      mask TypeOptions multiplier_implementation: behavioral HDL | standard core | embedded multiplier core
  bus_mul5 : Subsystem  AncestorBlock=casper_library_bus/bus_mult  mask(bus_mult){n_bits_a=[18 18 18 18 18 18 18 18 18 18 18 18 18 18 18 18], bin_pt_a=[16 16 16 16 16 16 16 16 16 16 16 16 16 16 16 16], type_a=[1 1 1 1 1 1 1 1 1 1 1 1 1 1 1 1], cmplx_a=off, n_bits_b=[8 8 8 8 8 8 8 8 8 8 8 8 8 8 8 8], bin_pt_b=[7 7 7 7 7 7 7 7 7 7 7 7 7 7 7 7], type_b=[1 1 1 1 1 1 1 1 1 1 1 1 1 1 1 1], cmplx_b=off, n_bits_out=[18 18 18 18 18 18 18 18 18 18 18 18 18 18 18 18], bin_pt_out=[16 16 16 16 16 16 16 16 16 16 16 16 16 16 16 16], type_out=[1 1 1 1 1 1 1 1 1 1 1 1 1 1 1 1], quantization=0, overflow=0, mult_latency=3, add_latency=1, conv_latency=1, max_fanout=2, fan_latency=0, multiplier_implementation=behavioral HDL, misc=off}
      mask prompts: n_bits_a "a input bit widths"; bin_pt_a "a input binary points"; type_a "a input type (Unsigned=0, Signed=1)"; cmplx_a "a input complex"; n_bits_b "b input bit widths"; bin_pt_b "b input binary points"; type_b "b input type (Unsigned=0, Signed=1)"; cmplx_b "b input complex"; n_bits_out "output bit widths"; bin_pt_out "output binary points"; type_out "output type (Unsigned=0, Signed=1)"; quantization "quantization strategy (Truncate=0, Round  (unbiased: +/- Inf)=1)"; overflow "overflow strategy (Wrap=0, Saturate=1, Flag as error=2)"; mult_latency "multiplier latency"; add_latency "adder latency"; conv_latency "convert latency"; max_fanout "limit fanout to ?"; fan_latency "fanout register latency"; multiplier_implementation "multiplier implementation"; misc "misc support"
      mask help: Multiply components of two busses
      mask init: same as r2daq_blocks/DigitalDownConverterExt/bus_mul_cosine
      mask TypeOptions multiplier_implementation: behavioral HDL | standard core | embedded multiplier core
  bus_mul6 : Subsystem  AncestorBlock=casper_library_bus/bus_mult  mask(bus_mult){n_bits_a=[18 18 18 18 18 18 18 18 18 18 18 18 18 18 18 18], bin_pt_a=[16 16 16 16 16 16 16 16 16 16 16 16 16 16 16 16], type_a=[1 1 1 1 1 1 1 1 1 1 1 1 1 1 1 1], cmplx_a=off, n_bits_b=[8 8 8 8 8 8 8 8 8 8 8 8 8 8 8 8], bin_pt_b=[7 7 7 7 7 7 7 7 7 7 7 7 7 7 7 7], type_b=[1 1 1 1 1 1 1 1 1 1 1 1 1 1 1 1], cmplx_b=off, n_bits_out=[18 18 18 18 18 18 18 18 18 18 18 18 18 18 18 18], bin_pt_out=[16 16 16 16 16 16 16 16 16 16 16 16 16 16 16 16], type_out=[1 1 1 1 1 1 1 1 1 1 1 1 1 1 1 1], quantization=0, overflow=0, mult_latency=3, add_latency=1, conv_latency=1, max_fanout=2, fan_latency=0, multiplier_implementation=behavioral HDL, misc=off}
      mask prompts: n_bits_a "a input bit widths"; bin_pt_a "a input binary points"; type_a "a input type (Unsigned=0, Signed=1)"; cmplx_a "a input complex"; n_bits_b "b input bit widths"; bin_pt_b "b input binary points"; type_b "b input type (Unsigned=0, Signed=1)"; cmplx_b "b input complex"; n_bits_out "output bit widths"; bin_pt_out "output binary points"; type_out "output type (Unsigned=0, Signed=1)"; quantization "quantization strategy (Truncate=0, Round  (unbiased: +/- Inf)=1)"; overflow "overflow strategy (Wrap=0, Saturate=1, Flag as error=2)"; mult_latency "multiplier latency"; add_latency "adder latency"; conv_latency "convert latency"; max_fanout "limit fanout to ?"; fan_latency "fanout register latency"; multiplier_implementation "multiplier implementation"; misc "misc support"
      mask help: Multiply components of two busses
      mask init: same as r2daq_blocks/DigitalDownConverterExt/bus_mul_cosine
      mask TypeOptions multiplier_implementation: behavioral HDL | standard core | embedded multiplier core
  bus_mul7 : Subsystem  AncestorBlock=casper_library_bus/bus_mult  mask(bus_mult){n_bits_a=[18 18 18 18 18 18 18 18 18 18 18 18 18 18 18 18], bin_pt_a=[16 16 16 16 16 16 16 16 16 16 16 16 16 16 16 16], type_a=[1 1 1 1 1 1 1 1 1 1 1 1 1 1 1 1], cmplx_a=off, n_bits_b=[8 8 8 8 8 8 8 8 8 8 8 8 8 8 8 8], bin_pt_b=[7 7 7 7 7 7 7 7 7 7 7 7 7 7 7 7], type_b=[1 1 1 1 1 1 1 1 1 1 1 1 1 1 1 1], cmplx_b=off, n_bits_out=[18 18 18 18 18 18 18 18 18 18 18 18 18 18 18 18], bin_pt_out=[16 16 16 16 16 16 16 16 16 16 16 16 16 16 16 16], type_out=[1 1 1 1 1 1 1 1 1 1 1 1 1 1 1 1], quantization=0, overflow=0, mult_latency=3, add_latency=1, conv_latency=1, max_fanout=2, fan_latency=0, multiplier_implementation=behavioral HDL, misc=off}
      mask prompts: n_bits_a "a input bit widths"; bin_pt_a "a input binary points"; type_a "a input type (Unsigned=0, Signed=1)"; cmplx_a "a input complex"; n_bits_b "b input bit widths"; bin_pt_b "b input binary points"; type_b "b input type (Unsigned=0, Signed=1)"; cmplx_b "b input complex"; n_bits_out "output bit widths"; bin_pt_out "output binary points"; type_out "output type (Unsigned=0, Signed=1)"; quantization "quantization strategy (Truncate=0, Round  (unbiased: +/- Inf)=1)"; overflow "overflow strategy (Wrap=0, Saturate=1, Flag as error=2)"; mult_latency "multiplier latency"; add_latency "adder latency"; conv_latency "convert latency"; max_fanout "limit fanout to ?"; fan_latency "fanout register latency"; multiplier_implementation "multiplier implementation"; misc "misc support"
      mask help: Multiply components of two busses
      mask init: same as r2daq_blocks/DigitalDownConverterExt/bus_mul_cosine
      mask TypeOptions multiplier_implementation: behavioral HDL | standard core | embedded multiplier core
  sync_mul_delay : xbsIndex_r4/Delay  rst=off  infoeditControl=Selection of Reset will increase slice count due to use of real FFs and instead of SRLs  en=off  latency=3  dbl_ovrd=off  reg_retiming=off  block_type=delay
  term{1..7} (7 alike) : Terminator
  sync_out : Outport
  y : Outport  Port=2
  wires:
  sync_in/1 -> sync_mul_delay/1
  sync_mul_delay/1 -> [gt_sync_in]
  data/1 -> [gt_data]
  cb0/1 -> [gt_cb0]
  cb1/1 -> [gt_cb1]
  cb2/1 -> [gt_cb2]
  cb3/1 -> [gt_cb3]
  cb4/1 -> [gt_cb4]
  cb5/1 -> [gt_cb5]
  cb6/1 -> [gt_cb6]
  cb7/1 -> [gt_cb7]
  [gt_data] -> bus_mul0/1(a)
  [gt_cb0] -> bus_mul0/2(b)
  [gt_data] -> bus_del1/1(din)
  bus_del1/1(dout) -> bus_mul1/1(a)
  [gt_cb1] -> bus_mul1/2(b)
  [gt_data] -> bus_del2/1(din)
  bus_del2/1(dout) -> bus_mul2/1(a)
  [gt_cb2] -> bus_mul2/2(b)
  [gt_data] -> bus_del3/1(din)
  bus_del3/1(dout) -> bus_mul3/1(a)
  [gt_cb3] -> bus_mul3/2(b)
  [gt_data] -> bus_del4/1(din)
  bus_del4/1(dout) -> bus_mul4/1(a)
  [gt_cb4] -> bus_mul4/2(b)
  [gt_data] -> bus_del5/1(din)
  bus_del5/1(dout) -> bus_mul5/1(a)
  [gt_cb5] -> bus_mul5/2(b)
  [gt_data] -> bus_del6/1(din)
  bus_del6/1(dout) -> bus_mul6/1(a)
  [gt_cb6] -> bus_mul6/2(b)
  [gt_data] -> bus_del7/1(din)
  bus_del7/1(dout) -> bus_mul7/1(a)
  [gt_cb7] -> bus_mul7/2(b)
  bus_mul0/1(a*b) -> bus_exp0/1(bus_in)
  bus_mul1/1(a*b) -> bus_exp1/1(bus_in)
  bus_mul2/1(a*b) -> bus_exp2/1(bus_in)
  bus_mul3/1(a*b) -> bus_exp3/1(bus_in)
  bus_mul4/1(a*b) -> bus_exp4/1(bus_in)
  bus_mul5/1(a*b) -> bus_exp5/1(bus_in)
  bus_mul6/1(a*b) -> bus_exp6/1(bus_in)
  bus_mul7/1(a*b) -> bus_exp7/1(bus_in)
  bus_exp0/1(msb_out16) -> adder_tree0/2(din1)
  bus_exp0/2(out15) -> adder_tree0/3(din2)
  bus_exp0/3(out14) -> adder_tree0/4(din3)
  bus_exp0/4(out13) -> adder_tree0/5(din4)
  bus_exp0/5(out12) -> adder_tree0/6(din5)
  bus_exp0/6(out11) -> adder_tree0/7(din6)
  bus_exp0/7(out10) -> adder_tree0/8(din7)
  bus_exp0/8(out9) -> adder_tree0/9(din8)
  bus_exp0/9(out8) -> adder_tree0/10(din9)
  bus_exp0/10(out7) -> adder_tree0/11(din10)
  bus_exp0/11(out6) -> adder_tree0/12(din11)
  bus_exp0/12(out5) -> adder_tree0/13(din12)
  bus_exp0/13(out4) -> adder_tree0/14(din13)
  bus_exp0/14(out3) -> adder_tree0/15(din14)
  bus_exp0/15(out2) -> adder_tree0/16(din15)
  bus_exp0/16(lsb_out1) -> adder_tree0/17(din16)
  [gt_sync_in] -> adder_tree0/1(sync)
  bus_exp1/1(msb_out16) -> adder_tree1/2(din1)
  bus_exp1/2(out15) -> adder_tree1/3(din2)
  bus_exp1/3(out14) -> adder_tree1/4(din3)
  bus_exp1/4(out13) -> adder_tree1/5(din4)
  bus_exp1/5(out12) -> adder_tree1/6(din5)
  bus_exp1/6(out11) -> adder_tree1/7(din6)
  bus_exp1/7(out10) -> adder_tree1/8(din7)
  bus_exp1/8(out9) -> adder_tree1/9(din8)
  bus_exp1/9(out8) -> adder_tree1/10(din9)
  bus_exp1/10(out7) -> adder_tree1/11(din10)
  bus_exp1/11(out6) -> adder_tree1/12(din11)
  bus_exp1/12(out5) -> adder_tree1/13(din12)
  bus_exp1/13(out4) -> adder_tree1/14(din13)
  bus_exp1/14(out3) -> adder_tree1/15(din14)
  bus_exp1/15(out2) -> adder_tree1/16(din15)
  bus_exp1/16(lsb_out1) -> adder_tree1/17(din16)
  [gt_sync_in] -> adder_tree1/1(sync)
  bus_exp2/1(msb_out16) -> adder_tree2/2(din1)
  bus_exp2/2(out15) -> adder_tree2/3(din2)
  bus_exp2/3(out14) -> adder_tree2/4(din3)
  bus_exp2/4(out13) -> adder_tree2/5(din4)
  bus_exp2/5(out12) -> adder_tree2/6(din5)
  bus_exp2/6(out11) -> adder_tree2/7(din6)
  bus_exp2/7(out10) -> adder_tree2/8(din7)
  bus_exp2/8(out9) -> adder_tree2/9(din8)
  bus_exp2/9(out8) -> adder_tree2/10(din9)
  bus_exp2/10(out7) -> adder_tree2/11(din10)
  bus_exp2/11(out6) -> adder_tree2/12(din11)
  bus_exp2/12(out5) -> adder_tree2/13(din12)
  bus_exp2/13(out4) -> adder_tree2/14(din13)
  bus_exp2/14(out3) -> adder_tree2/15(din14)
  bus_exp2/15(out2) -> adder_tree2/16(din15)
  bus_exp2/16(lsb_out1) -> adder_tree2/17(din16)
  [gt_sync_in] -> adder_tree2/1(sync)
  bus_exp3/1(msb_out16) -> adder_tree3/2(din1)
  bus_exp3/2(out15) -> adder_tree3/3(din2)
  bus_exp3/3(out14) -> adder_tree3/4(din3)
  bus_exp3/4(out13) -> adder_tree3/5(din4)
  bus_exp3/5(out12) -> adder_tree3/6(din5)
  bus_exp3/6(out11) -> adder_tree3/7(din6)
  bus_exp3/7(out10) -> adder_tree3/8(din7)
  bus_exp3/8(out9) -> adder_tree3/9(din8)
  bus_exp3/9(out8) -> adder_tree3/10(din9)
  bus_exp3/10(out7) -> adder_tree3/11(din10)
  bus_exp3/11(out6) -> adder_tree3/12(din11)
  bus_exp3/12(out5) -> adder_tree3/13(din12)
  bus_exp3/13(out4) -> adder_tree3/14(din13)
  bus_exp3/14(out3) -> adder_tree3/15(din14)
  bus_exp3/15(out2) -> adder_tree3/16(din15)
  bus_exp3/16(lsb_out1) -> adder_tree3/17(din16)
  [gt_sync_in] -> adder_tree3/1(sync)
  bus_exp4/1(msb_out16) -> adder_tree4/2(din1)
  bus_exp4/2(out15) -> adder_tree4/3(din2)
  bus_exp4/3(out14) -> adder_tree4/4(din3)
  bus_exp4/4(out13) -> adder_tree4/5(din4)
  bus_exp4/5(out12) -> adder_tree4/6(din5)
  bus_exp4/6(out11) -> adder_tree4/7(din6)
  bus_exp4/7(out10) -> adder_tree4/8(din7)
  bus_exp4/8(out9) -> adder_tree4/9(din8)
  bus_exp4/9(out8) -> adder_tree4/10(din9)
  bus_exp4/10(out7) -> adder_tree4/11(din10)
  bus_exp4/11(out6) -> adder_tree4/12(din11)
  bus_exp4/12(out5) -> adder_tree4/13(din12)
  bus_exp4/13(out4) -> adder_tree4/14(din13)
  bus_exp4/14(out3) -> adder_tree4/15(din14)
  bus_exp4/15(out2) -> adder_tree4/16(din15)
  bus_exp4/16(lsb_out1) -> adder_tree4/17(din16)
  [gt_sync_in] -> adder_tree4/1(sync)
  bus_exp5/1(msb_out16) -> adder_tree5/2(din1)
  bus_exp5/2(out15) -> adder_tree5/3(din2)
  bus_exp5/3(out14) -> adder_tree5/4(din3)
  bus_exp5/4(out13) -> adder_tree5/5(din4)
  bus_exp5/5(out12) -> adder_tree5/6(din5)
  bus_exp5/6(out11) -> adder_tree5/7(din6)
  bus_exp5/7(out10) -> adder_tree5/8(din7)
  bus_exp5/8(out9) -> adder_tree5/9(din8)
  bus_exp5/9(out8) -> adder_tree5/10(din9)
  bus_exp5/10(out7) -> adder_tree5/11(din10)
  bus_exp5/11(out6) -> adder_tree5/12(din11)
  bus_exp5/12(out5) -> adder_tree5/13(din12)
  bus_exp5/13(out4) -> adder_tree5/14(din13)
  bus_exp5/14(out3) -> adder_tree5/15(din14)
  bus_exp5/15(out2) -> adder_tree5/16(din15)
  bus_exp5/16(lsb_out1) -> adder_tree5/17(din16)
  [gt_sync_in] -> adder_tree5/1(sync)
  bus_exp6/1(msb_out16) -> adder_tree6/2(din1)
  bus_exp6/2(out15) -> adder_tree6/3(din2)
  bus_exp6/3(out14) -> adder_tree6/4(din3)
  bus_exp6/4(out13) -> adder_tree6/5(din4)
  bus_exp6/5(out12) -> adder_tree6/6(din5)
  bus_exp6/6(out11) -> adder_tree6/7(din6)
  bus_exp6/7(out10) -> adder_tree6/8(din7)
  bus_exp6/8(out9) -> adder_tree6/9(din8)
  bus_exp6/9(out8) -> adder_tree6/10(din9)
  bus_exp6/10(out7) -> adder_tree6/11(din10)
  bus_exp6/11(out6) -> adder_tree6/12(din11)
  bus_exp6/12(out5) -> adder_tree6/13(din12)
  bus_exp6/13(out4) -> adder_tree6/14(din13)
  bus_exp6/14(out3) -> adder_tree6/15(din14)
  bus_exp6/15(out2) -> adder_tree6/16(din15)
  bus_exp6/16(lsb_out1) -> adder_tree6/17(din16)
  [gt_sync_in] -> adder_tree6/1(sync)
  bus_exp7/1(msb_out16) -> adder_tree7/2(din1)
  bus_exp7/2(out15) -> adder_tree7/3(din2)
  bus_exp7/3(out14) -> adder_tree7/4(din3)
  bus_exp7/4(out13) -> adder_tree7/5(din4)
  bus_exp7/5(out12) -> adder_tree7/6(din5)
  bus_exp7/6(out11) -> adder_tree7/7(din6)
  bus_exp7/7(out10) -> adder_tree7/8(din7)
  bus_exp7/8(out9) -> adder_tree7/9(din8)
  bus_exp7/9(out8) -> adder_tree7/10(din9)
  bus_exp7/10(out7) -> adder_tree7/11(din10)
  bus_exp7/11(out6) -> adder_tree7/12(din11)
  bus_exp7/12(out5) -> adder_tree7/13(din12)
  bus_exp7/13(out4) -> adder_tree7/14(din13)
  bus_exp7/14(out3) -> adder_tree7/15(din14)
  bus_exp7/15(out2) -> adder_tree7/16(din15)
  bus_exp7/16(lsb_out1) -> adder_tree7/17(din16)
  [gt_sync_in] -> adder_tree7/1(sync)
  adder_tree0/1(sync_out) -> adder_tree_global/1(sync)
  adder_tree0/2(dout) -> adder_tree_global/2(din1)
  adder_tree1/1(sync_out) -> term1/1
  adder_tree1/2(dout) -> adder_tree_global/3(din2)
  adder_tree2/1(sync_out) -> term2/1
  adder_tree2/2(dout) -> adder_tree_global/4(din3)
  adder_tree3/1(sync_out) -> term3/1
  adder_tree3/2(dout) -> adder_tree_global/5(din4)
  adder_tree4/1(sync_out) -> term4/1
  adder_tree4/2(dout) -> adder_tree_global/6(din5)
  adder_tree5/1(sync_out) -> term5/1
  adder_tree5/2(dout) -> adder_tree_global/7(din6)
  adder_tree6/1(sync_out) -> term6/1
  adder_tree6/2(dout) -> adder_tree_global/8(din7)
  adder_tree7/1(sync_out) -> term7/1
  adder_tree7/2(dout) -> adder_tree_global/9(din8)
  adder_tree_global/1(sync_out) -> sync_out/1
  adder_tree_global/2(dout) -> y/1
